simulink model "walkingRobot_step4_library"  (R2019b)
settings: Solver=ode15s  StartTime=0.0  StopTime=10  EnableMultiTasking=on
PreLoadFcn:
  | robotParameters
  | load jointAngs
libraries: walkingRobotUtils x3
settings Model: Creator=bkim  LastModifiedBy=scastro
settings DataIOCC: ReturnWorkspaceOutputs=off  OutputSaveName=simout  OutputTimes=0:0.01:10
settings OptimizationCC: LifeSpan=inf
settings DebuggingCC: AllowSymbolicDim=off  PregeneratedLibrarySubsystemCodeDiagnostic=none  SFUnexpectedBacktrackingDiag=warning  SFNoUnconditionalDefaultTransitionDiag=warning  SFExecutionAtInitializationDiag=none  UnitsInconsistencyMsg=none  ArithmeticOperatorsInVariantConditions=warning
settings SFSimCC: SimUseLocalCustomCode=off  CustomCodeUndefinedFunction=UseInterfaceOnly
settings RTWCC: RTWUseLocalCustomCode=off
settings CodeAppCC: StateflowObjectComments=on
settings GRTTargetCC: TargetLangStandard=C89/C90 (ANSI)  GeneratePreprocessorConditionals=Disable all
settings ConfigComp: CovMetricSettings=dw  CovHtmlReporting=on  CovSaveCumulativeToWorkspaceVar=on  CovSaveSingleToWorkspaceVar=on  CovExternalEMLEnable=off  CovSFcnEnable=off
settings SimscapeCC: SimscapeNormalizeSystem=off  SimscapeLogOpenViewer=on  SimscapeLogLimitData=off  SimscapeLogDataHistory=10000
settings ConfigurationSet: Description=SimMechanics 2G
settings DiagnosticsConfigSet: SimMechanicsRigidlyBoundBlock=none
settings ExplorerConfigSet: InternalSimMechanicsExplorerSettings="<ExplorerConfiguration><canonicalview>default</canonicalview><AnimationSetting><BasePlaybackSpeed>1.0</BasePlaybackSpeed><PlaybackSpeedFactor>1.0</PlaybackSpeedFactor></AnimationSetting><TilePanel><TileInfo><Tiles Columns=\"1\" Count=\"1\" Rows=\"1\"><Column Weight=\"1\"/><Row Weight=\"1\"/><Tile Height=\"1\" Width=\"1\" X=\"0\" Y=\"0\"/></Tiles></TileInfo><SceneInfo><SceneViewer><BGColor><R>0.60000002384185791</R><G>0.60000002384185791</G><B>0.60000002384185791</B></BGColor><Camera><DoPerspective>off</DoPerspective><Position><X>-8.743766578094327</X><Y>22.8655522039700649</Y><Z>7.34244463036883044</Z></Position><Center><X>-0.694107743695583035</X><Y>0.447627991616262655</Y><Z>-0.726319279811428076</Z></Center><Up><X>0.189286953589408086</X><Y>-0.271655780544975634</Y><Z>0.943596092667483233</Z></Up><ViewLimDist>1</ViewLimDist><YLim>2.37101751638528224</YLim><XLim>3.03695144845645704</XLim></Camera></SceneViewer></SceneInfo></TilePanel><MechEditorPanel><Cameras/><GfxPanelCameraMap/><VideoCreator><PlaybackSpeedRatio>1.0</PlaybackSpeedRatio><FrameRate>30</FrameRate><VideoFormat>Motion JPEG AVI</VideoFormat><FrameSize>auto</FrameSize></VideoCreator></MechEditorPanel></ExplorerConfiguration>"

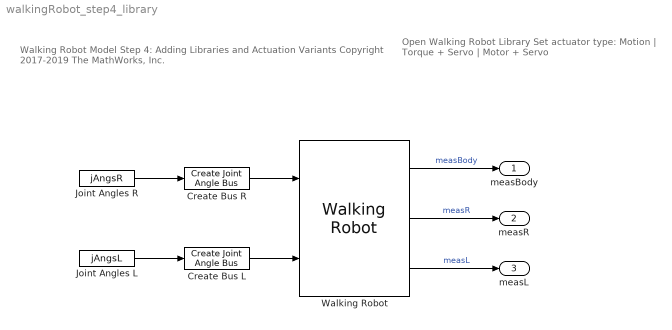
== system walkingRobot_step4_library ==
  note: Walking Robot Model
      | Step 4: Adding Libraries and Actuation Variants
      |
      | Copyright 2017-2019 The MathWorks, Inc.
  note: Open Walking Robot Library
      |
      | Set actuator type:
      | Motion | Torque + Servo | Motor + Servo
  Create Bus L : walkingRobotUtils/Create Joint Angle Bus  SystemSampleTime=-1  Latency=0  AutoFrameSizeCalculation=off
  Create Bus R : walkingRobotUtils/Create Joint Angle Bus  SystemSampleTime=-1  Latency=0  AutoFrameSizeCalculation=off
  Joint Angles L : FromWorkspace  VariableName=jAngsL  SampleTime=0  OutputAfterFinalValue=Holding final value
  Joint Angles R : FromWorkspace  VariableName=jAngsR  SampleTime=0  OutputAfterFinalValue=Holding final value
  Walking Robot : walkingRobotUtils/Walking Robot  SystemSampleTime=-1  Latency=0  AutoFrameSizeCalculation=off
  measBody : Outport  VectorParamsAs1DForOutWhenUnconnected=off
  measR : Outport  Port=2  VectorParamsAs1DForOutWhenUnconnected=off
  measL : Outport  Port=3  VectorParamsAs1DForOutWhenUnconnected=off
  wires:
  Walking Robot/3 -> measL/1  "measL"
  Walking Robot/2 -> measR/1  "measR"
  Create Bus R/1 -> Walking Robot/1
  Create Bus L/1 -> Walking Robot/2
  Joint Angles R/1 -> Create Bus R/1
  Joint Angles L/1 -> Create Bus L/1
  Walking Robot/1 -> measBody/1  "measBody"
